simulink model "Modell1"  (R2022b)
settings: Solver=VariableStepAuto  StartTime=0.0  StopTime=10.0  RelTol=1e-3
settings Model: Creator=bornk  LastModifiedBy=bornk

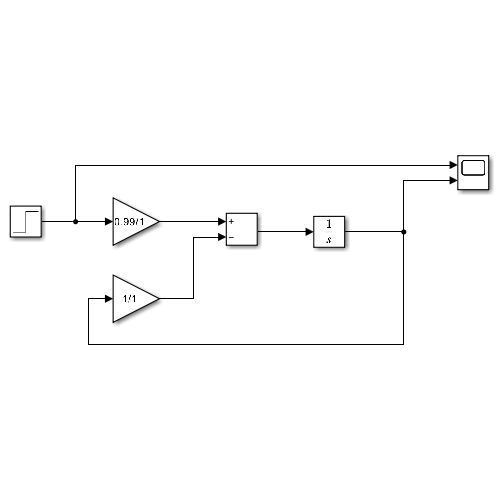
[thumbnail: Simulink's stored preview of the top-level diagram]
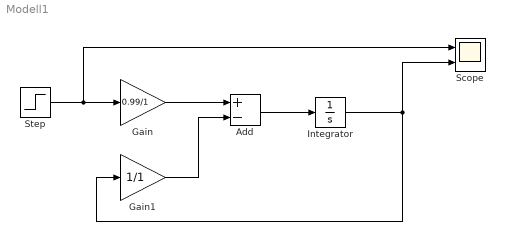
== system Modell1 ==
  Add : Sum  Inputs=+-
  Gain : Gain  Gain=0.99/1
  Gain1 : Gain  Gain=1/1
  Integrator : Integrator
  Scope : Scope  NumInputPorts=2
  Step : Step  SampleTime=0
  wires:
  Integrator/1 -> Scope/2, Gain1/1
  Add/1 -> Integrator/1
  Gain/1 -> Add/1
  Step/1 -> Scope/1, Gain/1
  Gain1/1 -> Add/2
